simulink model "my_model"  (R2024b)
settings: Solver=FixedStepAuto  StartTime=0.0  StopTime=10.0  RelTol=1e-3
undefined symbols (not defined in the file or in its folder): recurrentNet
libraries: dlutilitylib x2, dlconvfclib x2, dlsequencelib x2, dlactivationlib x1
settings Model: Creator=sebahattin.babur  LastModifiedBy=sebahattin.babur
settings OptimizationCC: DefaultParameterBehavior=Inlined  EnhancedBackFolding=on  PassReuseOutputArgsAs=Individual arguments  ZeroExternalMemoryAtStartup=off  ZeroInternalMemoryAtStartup=off  OptimizeBlockOrder=speed  DifferentSizesBufferReuse=on  OptimizationCustomize=off  EfficientTunableParamExpr=on
settings DebuggingCC: ParameterTunabilityLossMsg=error
settings SFSimCC: MATLABDynamicMemAlloc=off
settings RTWCC: Description=Embedded Coder  SystemTargetFile=ert.tlc  TemplateMakefile=ert_default_tmf
settings CodeAppCC: ForceParamTrailComments=on  IgnoreCustomStorageClasses=off  OperatorAnnotations=on  SimulinkDataObjDesc=on  SFDataObjDesc=on  InsertBlockDesc=on
settings ERTTargetCC: TargetLangStandard=C99 (ISO)  GenerateSampleERTMain=on  ERTCustomFileTemplate=example_file_process.tlc

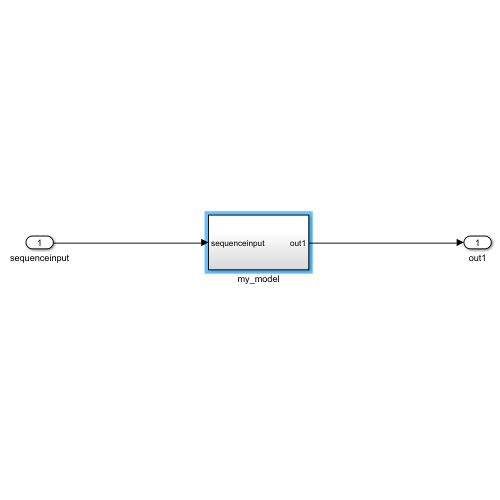
[thumbnail: Simulink's stored preview of the top-level diagram]
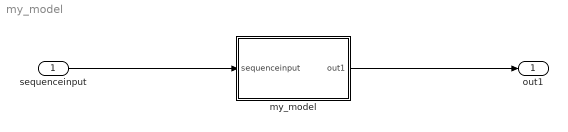
== system my_model ==
  sequenceinput : Inport  PortDimensions="[3  1]"
  my_model : Subsystem
  out1 : Outport
  wires:
  sequenceinput/1 -> my_model/1(sequenceinput)
  my_model/1(out1) -> out1/1

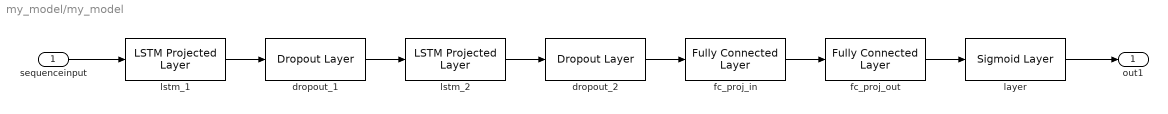
== system my_model/my_model ==
  sequenceinput : Inport  PortDimensions="[3  1]"
  dropout_1 : dlutilitylib/Dropout Layer  SampleTime=-1
  dropout_2 : dlutilitylib/Dropout Layer  SampleTime=-1
  fc_proj_in : dlconvfclib/Fully Connected Layer  Layer=recurrentNet.Layers(6)  OutMin=[]  OutMax=[]  WeightsDataTypeStr=Inherit: Inherit via back propagation  WeightsMin=[]  WeightsMax=[]  BiasDataTypeStr=Inherit: Inherit via back propagation  BiasMin=[]  BiasMax=[]  MatrixMultiplyMin=[]  MatrixMultiplyMax=[]  SampleTime=-1
      settings: DataFormat=CT
  fc_proj_out : dlconvfclib/Fully Connected Layer  Layer=recurrentNet.Layers(7)  OutMin=[]  OutMax=[]  WeightsDataTypeStr=Inherit: Inherit via back propagation  WeightsMin=[]  WeightsMax=[]  BiasDataTypeStr=Inherit: Inherit via back propagation  BiasMin=[]  BiasMax=[]  MatrixMultiplyMin=[]  MatrixMultiplyMax=[]  SampleTime=-1
      settings: DataFormat=CT
  layer : dlactivationlib/Sigmoid Layer  ApproximationMethod=None  OutMin=[]  OutMax=[]  SampleTime=-1
  lstm_1 : dlsequencelib/LSTM Projected Layer  Layer=recurrentNet.Layers(2)  Stateful=on  ApproximationMethod=None  InputWeightsDataTypeStr=Inherit: Inherit via back propagation  InputWeightsMin=[]  InputWeightsMax=[]  RecurrentWeightsDataTypeStr=Inherit: Inherit via back propagation  RecurrentWeightsMin=[]  RecurrentWeightsMax=[]  BiasDataTypeStr=Inherit: Inherit via back propagation  BiasMin=[]  BiasMax=[]  InputProjectorWeightsDataTypeStr=Inherit: Inherit via back propagation  InputProjectorWeightsMin=[]  InputProjectorWeightsMax=[]  OutputProjectorWeightsDataTypeStr=Inherit: Inherit via back propagation  OutputProjectorWeightsMin=[]  OutputProjectorWeightsMax=[]  InitialCellStateDataTypeStr=Inherit: Inherit via back propagation  InitialCellStateMin=[]  InitialCellStateMax=[]  CellStateMin=[]  CellStateMax=[]  InitialHiddenStateDataTypeStr=Inherit: Inherit via back propagation  InitialHiddenStateMin=[]  InitialHiddenStateMax=[]  HiddenStateMin=[]  HiddenStateMax=[]  InputWeightsMatrixMultiplyOutMin=[]  InputWeightsMatrixMultiplyOutMax=[]  RecurrentWeightsMatrixMultiplyOutMin=[]  RecurrentWeightsMatrixMultiplyOutMax=[]  InputProjectorWeightsMatrixMultiplyOutMin=[]  InputProjectorWeightsMatrixMultiplyOutMax=[]  OutputProjectorWeightsMatrixMultiplyOutMin=[]  OutputProjectorWeightsMatrixMultiplyOutMax=[]  LinearGateAddOutMin=[]  LinearGateAddOutMax=[]  CellStateProductOutMin=[]  CellStateProductOutMax=[]  SampleTime=-1
      settings: DataFormat=CT
  lstm_2 : dlsequencelib/LSTM Projected Layer  Layer=recurrentNet.Layers(4)  Stateful=on  ApproximationMethod=None  InputWeightsDataTypeStr=Inherit: Inherit via back propagation  InputWeightsMin=[]  InputWeightsMax=[]  RecurrentWeightsDataTypeStr=Inherit: Inherit via back propagation  RecurrentWeightsMin=[]  RecurrentWeightsMax=[]  BiasDataTypeStr=Inherit: Inherit via back propagation  BiasMin=[]  BiasMax=[]  InputProjectorWeightsDataTypeStr=Inherit: Inherit via back propagation  InputProjectorWeightsMin=[]  InputProjectorWeightsMax=[]  OutputProjectorWeightsDataTypeStr=Inherit: Inherit via back propagation  OutputProjectorWeightsMin=[]  OutputProjectorWeightsMax=[]  InitialCellStateDataTypeStr=Inherit: Inherit via back propagation  InitialCellStateMin=[]  InitialCellStateMax=[]  CellStateMin=[]  CellStateMax=[]  InitialHiddenStateDataTypeStr=Inherit: Inherit via back propagation  InitialHiddenStateMin=[]  InitialHiddenStateMax=[]  HiddenStateMin=[]  HiddenStateMax=[]  InputWeightsMatrixMultiplyOutMin=[]  InputWeightsMatrixMultiplyOutMax=[]  RecurrentWeightsMatrixMultiplyOutMin=[]  RecurrentWeightsMatrixMultiplyOutMax=[]  InputProjectorWeightsMatrixMultiplyOutMin=[]  InputProjectorWeightsMatrixMultiplyOutMax=[]  OutputProjectorWeightsMatrixMultiplyOutMin=[]  OutputProjectorWeightsMatrixMultiplyOutMax=[]  LinearGateAddOutMin=[]  LinearGateAddOutMax=[]  CellStateProductOutMin=[]  CellStateProductOutMax=[]  SampleTime=-1
      settings: DataFormat=CT
  out1 : Outport
  wires:
  lstm_1/1 -> dropout_1/1
  fc_proj_out/1 -> layer/1
  layer/1 -> out1/1
  dropout_2/1 -> fc_proj_in/1
  sequenceinput/1 -> lstm_1/1
  fc_proj_in/1 -> fc_proj_out/1
  dropout_1/1 -> lstm_2/1
  lstm_2/1 -> dropout_2/1
